simulink model "discrete_model_3_2_1"  (R2024b)
settings: Solver=ode5  StartTime=0.0  StopTime=20  FixedStep=0.001  RelTol=1e-3
undefined symbols (not defined in the file): Gam_o, H_o, J_o, K, National_Instruments, Nu, Nx, PCI, Phi_o, rpm2rads, sens, step_gain, T, u_bar_max
libraries: sldrtlib x3
settings Model: SimulationMode=external  ExtModeTrigDuration=20001  Creator=fasoloandr  LastModifiedBy=Enrico
settings DataIOCC: ReturnWorkspaceOutputs=off
settings HardwareCC: ProdBitPerLong=64  ProdHWDeviceType=Intel->x86-64 (Linux 64)
settings RTWCC: Description=Simulink Desktop Real-Time  SystemTargetFile=sldrt.tlc  TemplateMakefile=sldrt.tmf  RTWCompilerOptimization=on
settings CodeAppCC: MaxIdLength=95
settings SimulinkDesktopRealTimeCC: TargetLibSuffix=_sldrt.a  TargetPreCompLibLocation=D:\Programmi (D)\MATLAB\R2024b\toolbox\sldrt\lib\win64  ParMdlRefBuildCompliant=on

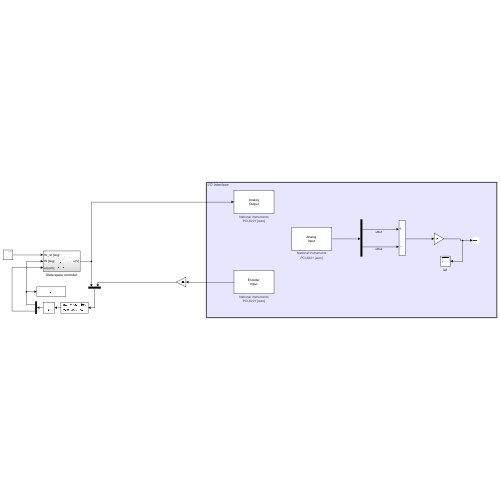
[thumbnail: Simulink's stored preview of the top-level diagram]
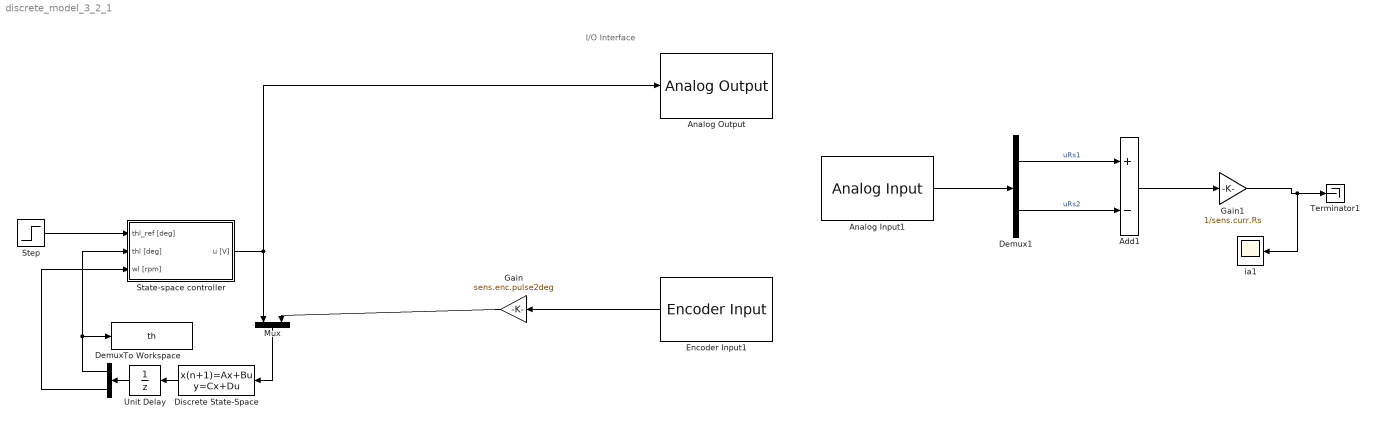
== system discrete_model_3_2_1 ==
  note: I/O Interface
  Add1 : Sum  Inputs=+-
  Analog Input1 : sldrtlib/Analog Input  SampleTime=-1  MaxMissedTicks=10  ShowMissedTicks=off  YieldWhenWaiting=off  DrvName=National_Instruments/PCI-6221  DrvAddress=4294967295  DrvOptions=[0 0 0 2 0]  Channels=[1,2]  RangeMode=1  VoltRange=1  DataType=1
      settings: AttributesFormatString=National Instruments\nPCI-6221 [auto]
  Analog Output : sldrtlib/Analog Output  SampleTime=-1  MaxMissedTicks=10  ShowMissedTicks=off  YieldWhenWaiting=off  DrvName=National_Instruments/PCI-6221  DrvAddress=4294967295  DrvOptions=[0 0 0 2 0]  Channels=1  RangeMode=1  VoltRange=1  InitialValue=[0]  FinalValue=[0]
      settings: AttributesFormatString=National Instruments\nPCI-6221 [auto]
  Demux : Demux  Outputs=2
  Demux1 : Demux  Outputs=2
  Discrete State-Space : DiscreteStateSpace  A=Phi_o  B=Gam_o  C=H_o  D=J_o  SampleTime=T
  Encoder Input1 : sldrtlib/Encoder Input  SampleTime=-1  MaxMissedTicks=10  ShowMissedTicks=off  YieldWhenWaiting=off  DrvName=National_Instruments/PCI-6221  DrvAddress=4294967295  DrvOptions=[0 0 0 2 0]  Channels=1  QuadMode=3  IndexPulse=1  InputFilter=Inf  DataType=1
      settings: AttributesFormatString=National Instruments\nPCI-6221 [auto]
  Gain : Gain  Gain=sens.enc.pulse2deg
  Gain1 : Gain  Gain=1/sens.curr.Rs
  Mux : Mux  Inputs=2
  State-space controller : Subsystem
  Step : Step  After=step_gain  SampleTime=0
  Terminator1 : Terminator
  To Workspace : ToWorkspace  VariableName=th  SaveFormat=Structure With Time  SampleTime=-1
  Unit Delay : UnitDelay  SampleTime=T  HasFrameUpgradeWarning=on
  ia1 : Scope
  wires:
  Gain1/1 -> ia1/1, Terminator1/1
  Demux1/1 -> Add1/1  "uRs1"
  Analog Input1/1 -> Demux1/1
  Demux1/2 -> Add1/2  "uRs2"
  Encoder Input1/1 -> Gain/1
  Add1/1 -> Gain1/1
  State-space controller/1(u [V]) -> Analog Output/1, Mux/1
  Demux/2 -> State-space controller/3(wl [rpm])
  Mux/1 -> Discrete State-Space/1
  Gain/1 -> Mux/2
  Demux/1 -> To Workspace/1, State-space controller/2(thl [deg])
  Step/1 -> State-space controller/1(thl_ref [deg])
  Unit Delay/1 -> Demux/1
  Discrete State-Space/1 -> Unit Delay/1

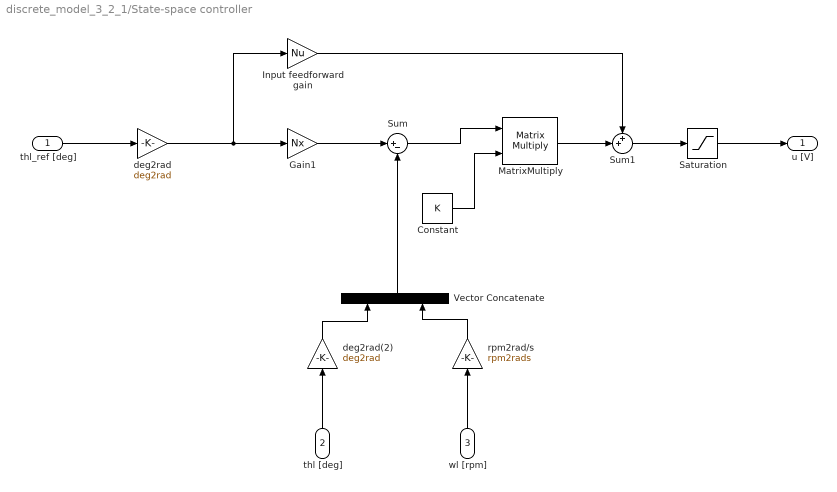
== system discrete_model_3_2_1/State-space controller ==
  thl_ref [deg] : Inport
  thl [deg] : Inport  Port=2
  wl [rpm] : Inport  Port=3
  Constant : Constant  Value=K
  Gain1 : Gain  Gain=Nx
  Input feedforward gain : Gain  Gain=Nu
  MatrixMultiply : Product  Multiplication=Matrix(*)
  Saturation : Saturate  UpperLimit=u_bar_max  LowerLimit=-u_bar_max
  Sum : Sum  Inputs=|+-
  Sum1 : Sum  Inputs=++|
  Vector Concatenate : Concatenate
  deg2rad : Gain  Gain=deg2rad
  deg2rad(2) : Gain  Gain=deg2rad
  rpm2rad/s : Gain  Gain=rpm2rads
  u [V] : Outport
  wires:
  rpm2rad/s/1 -> Vector Concatenate/2
  Gain1/1 -> Sum/1
  Sum1/1 -> Saturation/1
  thl [deg]/1 -> deg2rad(2)/1
  deg2rad/1 -> Input feedforward gain/1, Gain1/1
  deg2rad(2)/1 -> Vector Concatenate/1
  thl_ref [deg]/1 -> deg2rad/1
  wl [rpm]/1 -> rpm2rad/s/1
  Input feedforward gain/1 -> Sum1/1
  Vector Concatenate/1 -> Sum/2
  Saturation/1 -> u [V]/1
  MatrixMultiply/1 -> Sum1/2
  Sum/1 -> MatrixMultiply/1
  Constant/1 -> MatrixMultiply/2
